simulink model "IMU_ExtendedKalmanFilter_model"  (R2015a)
settings: Solver=ode45  StartTime=0.0  StopTime=10.0  RelTol=1e-3
settings Model: Creator=hamada  LastModifiedBy=hamada

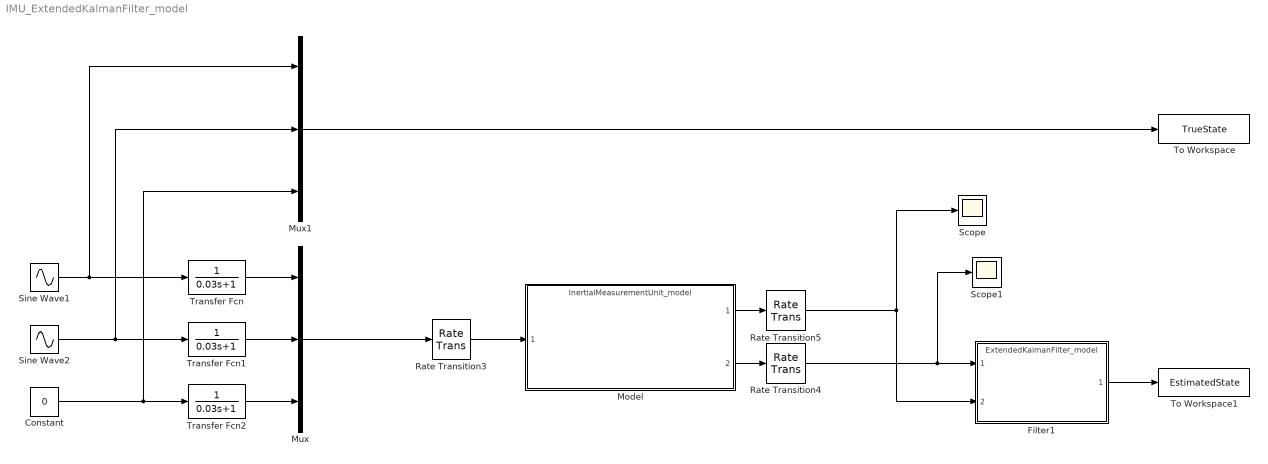
== system IMU_ExtendedKalmanFilter_model ==
  Constant : Constant  Value=0  SampleTime=0
  Filter1 : ModelReference  ModelNameDialog=ExtendedKalmanFilter_model.slx  SimulationMode=Normal  ModelReferenceVersion=1.50  CopyOfModelName=ExtendedKalmanFilter_model.slx  DefaultDataLogging=on
  Model : ModelReference  ModelNameDialog=InertialMeasurementUnit_model.slx  SimulationMode=Normal  ModelReferenceVersion=1.20  CopyOfModelName=InertialMeasurementUnit_model.slx  DefaultDataLogging=on
  Mux : Mux  Inputs=3
  Mux1 : Mux  Inputs=3
  Rate Transition3 : RateTransition
  Rate Transition4 : RateTransition
  Rate Transition5 : RateTransition
  Scope : Scope
  Scope1 : Scope
  Sine Wave1 : Sin  Amplitude=pi/6  SampleTime=0
  Sine Wave2 : Sin  Amplitude=pi/6  Phase=pi/2  SampleTime=0
  To Workspace : ToWorkspace  VariableName=TrueState  SaveFormat=Timeseries  SampleTime=-1
  To Workspace1 : ToWorkspace  VariableName=EstimatedState  SaveFormat=Timeseries  SampleTime=-1
  Transfer Fcn : TransferFcn  Denominator=[0.03 1]
  Transfer Fcn1 : TransferFcn  Denominator=[0.03 1]
  Transfer Fcn2 : TransferFcn  Denominator=[0.03 1]
  wires:
  Filter1/1 -> To Workspace1/1
  Model/1 -> Rate Transition5/1
  Model/2 -> Rate Transition4/1
  Mux/1 -> Rate Transition3/1
  Constant/1 -> Mux1/3, Transfer Fcn2/1
  Sine Wave1/1 -> Mux1/1, Transfer Fcn/1
  Sine Wave2/1 -> Mux1/2, Transfer Fcn1/1
  Rate Transition3/1 -> Model/1
  Rate Transition4/1 -> Scope1/1, Filter1/1
  Transfer Fcn/1 -> Mux/1
  Transfer Fcn1/1 -> Mux/2
  Transfer Fcn2/1 -> Mux/3
  Rate Transition5/1 -> Filter1/2, Scope/1
  Mux1/1 -> To Workspace/1
